simulink model "sb13_6c"  (Simulink 6.0)
settings: Solver=ode45  SolverMode=SingleTasking  StartTime=0.0  StopTime=999999  MaxStep=10  RelTol=1e-3  AbsTol=1e-6
values from neighbouring files (symbols this model uses):
  Gs = 10/(60*s+1)/(.1*s+1)    [m0108d.m]    (also in m0109b.m = 1/(8*s+1)^3; m0113c.m = 180/(.2*s+1)^3; m0251.m = b0/(a2*s^2+a1*s+a0); m0252.m = b0/(a2*s^2+a1*s+a0))
  Tsoll = 100    [m0113c.m]
settings Model: LastModifiedBy=Froriep
settings DataIOCC: LimitDataPoints=off  SaveOutput=off  SaveTime=off
settings OptimizationCC: BooleanDataType=off
settings DebuggingCC: SolverPrmCheckMsg=none
settings HardwareCC: TargetUnknown=on

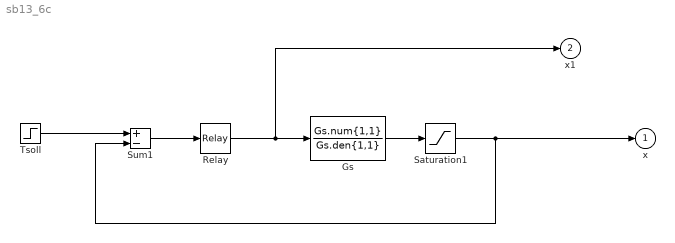
== system sb13_6c ==
  Gs : TransferFcn  Numerator=Gs.num{1,1}  Denominator=Gs.den{1,1}
  Relay : Relay  OnSwitchValue=100  OffSwitchValue=0  SampleTime=0
  Saturation1 : Saturate  UpperLimit=Tsoll  LowerLimit=-1000000
  Sum1 : Sum  Inputs=+-  SaturateOnIntegerOverflow=on  InputSameDT=on
  Tsoll : Step  Time=.1  After=Tsoll  SampleTime=0
  x : Outport  InitialOutput=0
  x1 : Outport  Port=2  InitialOutput=0
  wires:
  Tsoll/1 -> Sum1/1
  Gs/1 -> Saturation1/1
  Sum1/1 -> Relay/1
  Relay/1 -> Gs/1, x1/1
  Saturation1/1 -> Sum1/2, x/1
